simulink model "DYC_test"  (R2021b)
settings: Solver=ode4  StartTime=0.0  StopTime=1  FixedStep=0.001  RelTol=1e-3
values from neighbouring files (symbols this model uses):
  df = 1.225    [VehicleParamsFEM20.m]    (also in VehicleParamsFEM20_Gear17.m; VehicleParamsFEM21.m)
  lf = l*(1-WBf)    (= 0.7956)    [VehicleParamsFEM20.m]    (also in VehicleParamsFEM20_Gear17.m; VehicleParamsFEM21.m)
libraries: simulink x1
settings Model: Creator=tsuyoshi  LastModifiedBy=tsuyoshi

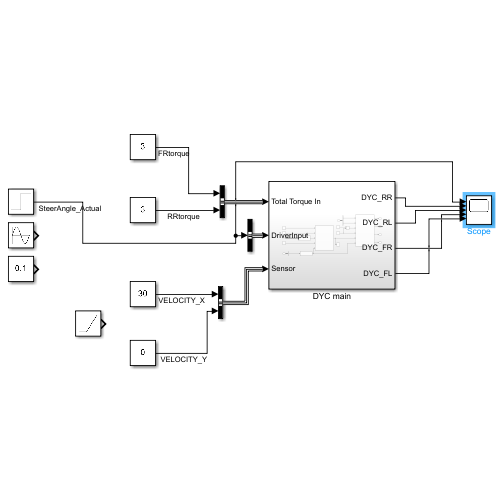
[thumbnail: Simulink's stored preview of the top-level diagram]
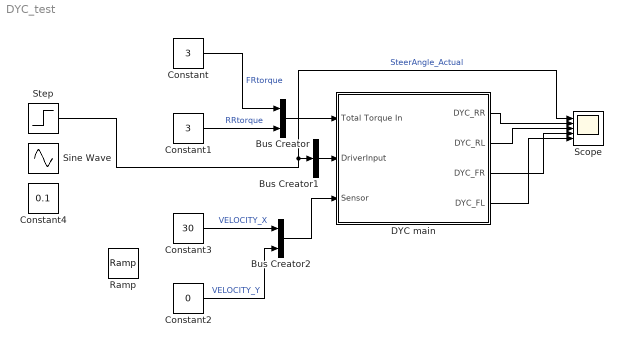
== system DYC_test ==
  Bus Creator : BusCreator  Inputs=2
  Bus Creator1 : BusCreator  Inputs=1
  Bus Creator2 : BusCreator  Inputs=2
  Constant : Constant  Value=3
  Constant1 : Constant  Value=3
  Constant2 : Constant  Value=0
  Constant3 : Constant  Value=30
  Constant4 : Constant  Value=0.1
  DYC main : Subsystem
  Ramp : simulink/Sources/Ramp  slope=10  start=0  InitialOutput=0
  Scope : Scope  NumInputPorts=5
  Sine Wave : Sin  Amplitude=0.2  Frequency=2*pi*1  SampleTime=0
  Step : Step  Time=0.2  After=0.1  SampleTime=0
  wires:
  DYC main/1(DYC_RR) -> Scope/2
  DYC main/2(DYC_RL) -> Scope/3
  DYC main/3(DYC_FR) -> Scope/4
  DYC main/4(DYC_FL) -> Scope/5
  Constant/1 -> Bus Creator/1  "FRtorque"
  Constant1/1 -> Bus Creator/2  "RRtorque"
  Bus Creator/1 -> DYC main/1(Total Torque In)
  Step/1 -> Scope/1, Bus Creator1/1  "SteerAngle_Actual"
  Bus Creator1/1 -> DYC main/2(DriverInput)
  Bus Creator2/1 -> DYC main/3(Sensor)
  Constant2/1 -> Bus Creator2/2  "VELOCITY_Y"
  Constant3/1 -> Bus Creator2/1  "VELOCITY_X"

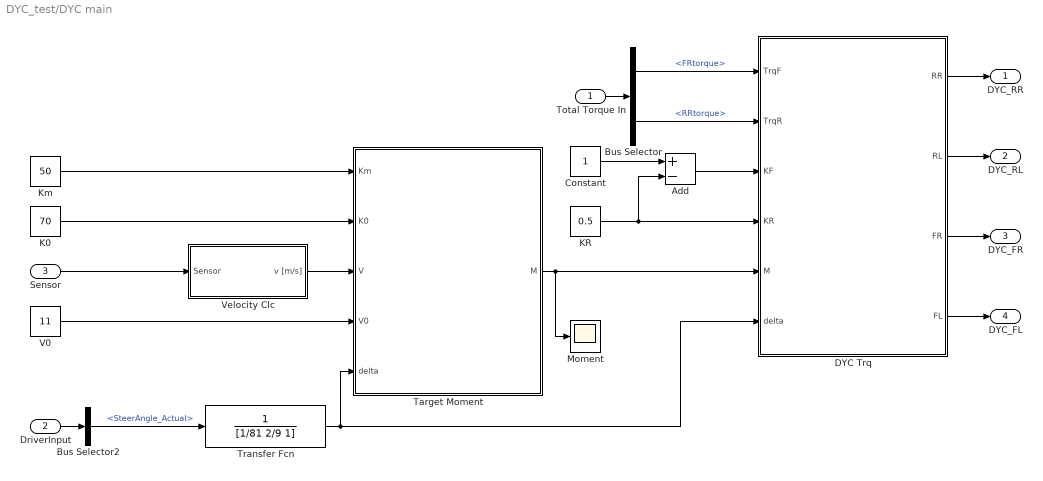
== system DYC_test/DYC main ==
  Total Torque In : Inport
  DriverInput : Inport  Port=2
  Sensor : Inport  Port=3
  Add : Sum  Inputs=+-
  Bus Selector : BusSelector  OutputSignals=FRtorque,RRtorque
  Bus Selector2 : BusSelector  OutputSignals=SteerAngle_Actual
  Constant : Constant
  DYC Trq : MATLAB Function  TreatAsAtomicUnit=on
  K0 : Constant  Value=70
  KR : Constant  Value=0.5
  Km : Constant  Value=50
  Moment : Scope
  Target Moment : MATLAB Function  TreatAsAtomicUnit=on
  Transfer Fcn : TransferFcn  Denominator=[1/81 2/9 1]
  V0 : Constant  Value=11
  Velocity Clc : Subsystem
  DYC_RR : Outport
  DYC_RL : Outport  Port=2
  DYC_FR : Outport  Port=3
  DYC_FL : Outport  Port=4
  wires:
  DriverInput/1 -> Bus Selector2/1
  Sensor/1 -> Velocity Clc/1(Sensor)
  Velocity Clc/1(v [m/s]) -> Target Moment/3(V)
  Km/1 -> Target Moment/1(Km)
  K0/1 -> Target Moment/2(K0)
  V0/1 -> Target Moment/4(V0)
  Bus Selector2/1 -> Transfer Fcn/1  "<SteerAngle_Actual>"
  Total Torque In/1 -> Bus Selector/1
  Bus Selector/1 -> DYC Trq/1(TrqF)  "<FRtorque>"
  Bus Selector/2 -> DYC Trq/2(TrqR)  "<RRtorque>"
  Add/1 -> DYC Trq/3(KF)
  KR/1 -> Add/2, DYC Trq/4(KR)
  Target Moment/1(M) -> DYC Trq/5(M), Moment/1
  Constant/1 -> Add/1
  DYC Trq/1(RR) -> DYC_RR/1
  DYC Trq/2(RL) -> DYC_RL/1
  DYC Trq/3(FR) -> DYC_FR/1
  DYC Trq/4(FL) -> DYC_FL/1
  Transfer Fcn/1 -> DYC Trq/6(delta), Target Moment/5(delta)

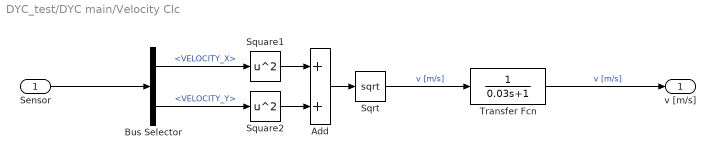
== system DYC_test/DYC main/Velocity Clc ==
  Sensor : Inport
  Add : Sum
  Bus Selector : BusSelector  OutputSignals=VELOCITY_X,VELOCITY_Y
  Sqrt : Sqrt  SaturateOnIntegerOverflow=on
  Square1 : Math  Operator=square  SaturateOnIntegerOverflow=on
  Square2 : Math  Operator=square  SaturateOnIntegerOverflow=on
  Transfer Fcn : TransferFcn  Denominator=[0.03 1]
  v [m/s] : Outport
  wires:
  Bus Selector/2 -> Square2/1  "<VELOCITY_Y>"
  Bus Selector/1 -> Square1/1  "<VELOCITY_X>"
  Add/1 -> Sqrt/1
  Square1/1 -> Add/1
  Sensor/1 -> Bus Selector/1
  Square2/1 -> Add/2
  Transfer Fcn/1 -> v [m/s]/1  "v [m/s]"
  Sqrt/1 -> Transfer Fcn/1  "v [m/s]"

== matlab function DYC_test/DYC main/Target Moment ==
  data: Km input; M output; K0 input; V input; V0 input; delta input
function M = fcn(Km, K0, V, V0, delta)
    if V<3/3.6
        M=0;
    else
        M=Km*(1+(K0/Km-1)*exp(-V/V0))*delta;
    end
end

== matlab function DYC_test/DYC main/DYC Trq ==
  data: RR output; RL output; FR output; TrqF input; TrqR input; KF input; KR input; M input; FL output; delta input; lf parameter; df parameter
function [RR, RL, FR, FL] = fcn(TrqF, TrqR, KF, KR, M, delta, lf, df)
    FL=(1+2*lf/df*tan(delta))*TrqF-(KF*M)/(df*cos(delta));
    FR=(1-2*lf/df*tan(delta))*TrqF+(KF*M)/(df*cos(delta));
    RL=TrqR-(KR*M)/df;
    RR=TrqR+(KR*M)/df;
end
